simulink model "m20p5"  (R2021b)
settings: Solver=ode45  StartTime=1  StopTime=10  FixedStep=0.1  RelTol=1e-3
undefined symbols (not defined in the file): seed61, seed62
settings Model: Creator=tanzc  LastModifiedBy=tanzc
settings DataIOCC: SaveFormat=Array  ReturnWorkspaceOutputs=off

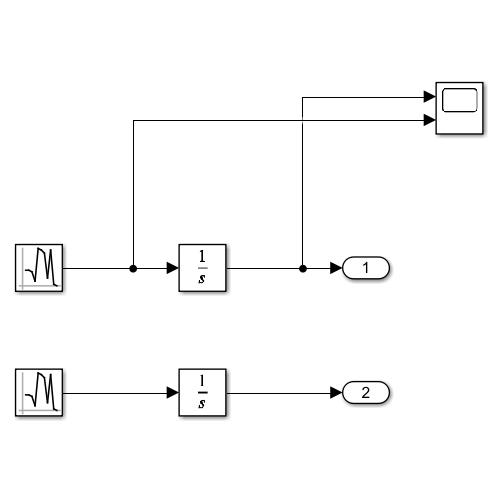
[thumbnail: Simulink's stored preview of the top-level diagram]
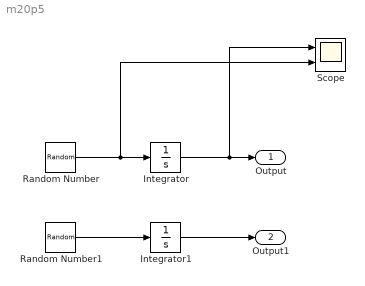
== system m20p5 ==
  Integrator : Integrator
  Integrator1 : Integrator
  Random Number : RandomNumber  Seed=seed61  SampleTime=0.1
  Random Number1 : RandomNumber  Seed=seed62  SampleTime=0.1
  Scope : Scope  NumInputPorts=2
  Output : Outport
  Output1 : Outport  Port=2
  wires:
  Random Number/1 -> Scope/2, Integrator/1
  Integrator/1 -> Scope/1, Output/1
  Random Number1/1 -> Integrator1/1
  Integrator1/1 -> Output1/1
